simulink model "zCtr"  (Simulink 7.9)
settings: Solver=ode45  StartTime=0.0  StopTime=15  RelTol=1e-3
undefined symbols (not defined in the file): satThrust, sigbuilder_block
libraries: simulink x2
settings Model: Creator=userk  LastModifiedBy=userk

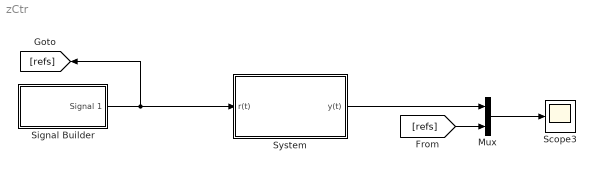
== system zCtr ==
  Mux : Mux  Inputs=2
  Scope3 : Scope
  Signal Builder : Subsystem  Tag=STV Subsys  LoadFcn=sigbuilder_block('load');  StartFcn=sigbuilder_block('start');  StopFcn=sigbuilder_block('stop');  ClipboardFcn=sigbuilder_block('clipboard');  mask(Sigbuilder block){}
      mask help: Simulink:masks:SigbuilderBlock_MD
      mask init:
      | if ~strcmp(get_param(bdroot(gcbh),'SimulationStatus'),'stopped') tuvar = sigbuilder_block('maskInit'); end
      settings: CopyFcn=sigbuilder_block('copy');  DeleteFcn=sigbuilder_block('delete');  ModelCloseFcn=sigbuilder_block('modelClose');  PreSaveFcn=sigbuilder_block('preSave');  PauseFcn=sigbuilder_block('pause');  ContinueFcn=sigbuilder_block('continue');  NameChangeFcn=sigbuilder_block('namechange');  OpenFcn=sigbuilder_block('open',[365.6 120.8 550.4 400 ]);  CloseFcn=sigbuilder_block('close');
      mask Display: plot(0, 0, 100, 100,[2, 2, 32, 32, 2], [68, 8, 8, 68, 68],[32, 2], [38, 38], [32, 19, 2],[53, 60, 44], [32, 17, 17, 2],[16, 16, 31, 31]);txt = getActiveGroup(gcbh);text(2, 100, txt,'verticalAlignment', 'top');
  System : Subsystem
  wires:
  Signal Builder/1(Signal 1) -> [refs], System/1(r(t))
  [refs] -> Mux/2
  Mux/1 -> Scope3/1
  System/1(y(t)) -> Mux/1

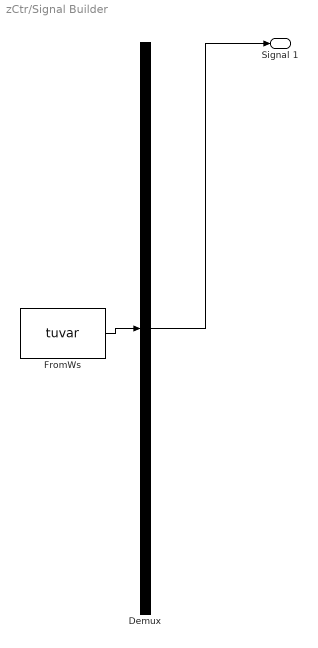
== system zCtr/Signal Builder ==
  Demux : Demux  Tag=STV Demux  Outputs=1
  FromWs : FromWorkspace  Tag=STV FromWs  VariableName=tuvar  SampleTime=0  SigBuilderData=DataTag0  VnvData=DataTag1
      SigBuilderData=|
      | common.afterFinalStr = 'Extrapolate'
      | common.sampleTime = 0
      | dataSet.timeRange = [0 10]
      | dataSet.name = 'Group 1'
      | sbobj.Groups.Name = 'Group 1'
      | sbobj.Groups.Signals.Name = 'Signal 1'
      | sbobj.Groups.Signals.XData = [0 4.06 4.06 6 6 10]
      | sbobj.Groups.Signals.YData = [0 0.995 1 1 0.995 0.01]
  Signal 1 : Outport  Tag=STV Outport
  wires:
  Demux/1 -> Signal 1/1
  FromWs/1 -> Demux/1

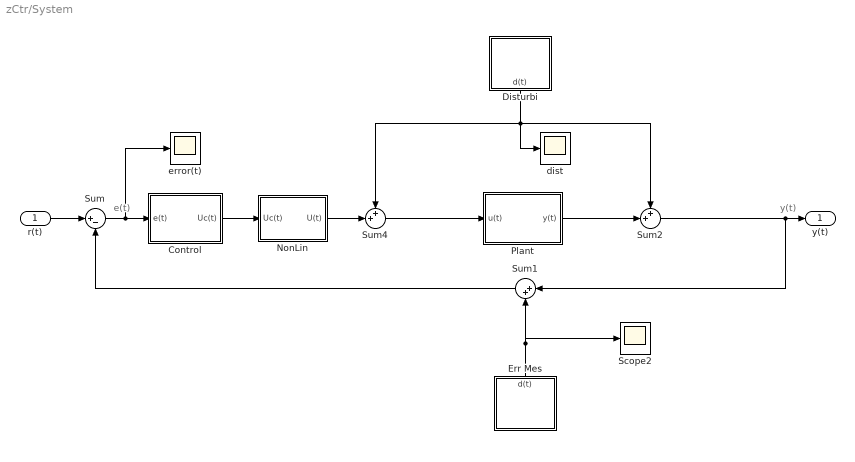
== system zCtr/System ==
  note: e(t)
  note: y(t)
  r(t) : Inport
  Control : Subsystem
  Disturbi : Subsystem
  Err Mes : Subsystem
  NonLin : Subsystem
  Plant : Subsystem
  Scope2 : Scope
      settings: SaveName=ScopeData2
  Sum : Sum  Inputs=|+-
  Sum1 : Sum  Inputs=|++
  Sum2 : Sum  Inputs=++|
  Sum4 : Sum  Inputs=++|
  dist : Scope
  error(t) : Scope
      settings: SaveName=ScopeData4
  y(t) : Outport
  wires:
  Sum/1 -> error(t)/1, Control/1(e(t))
  Plant/1(y(t)) -> Sum2/2
  Sum2/1 -> Sum1/1, y(t)/1
  Sum1/1 -> Sum/2
  Disturbi/1("  d(t)") -> dist/1, Sum4/1, Sum2/1
  Sum4/1 -> Plant/1(u(t))
  Control/1(Uc(t)) -> NonLin/1(Uc(t))
  NonLin/1(U(t)) -> Sum4/2
  r(t)/1 -> Sum/1
  Err Mes/1("  d(t)") -> Sum1/2, Scope2/1

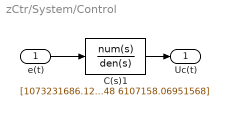
== system zCtr/System/Control ==
  e(t) : Inport
  C(s)1 : TransferFcn  Numerator=[1073231686.12918 1273486031.3238]  Denominator=[1 5043.9968441748 6107158.06951568]
  Uc(t) : Outport
  wires:
  e(t)/1 -> C(s)1/1
  C(s)1/1 -> Uc(t)/1

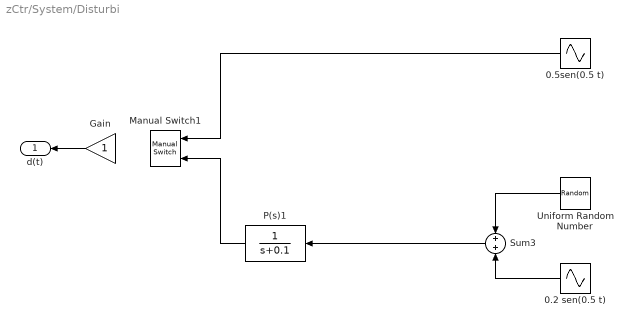
== system zCtr/System/Disturbi ==
  0.2 sen(0.5 t) : Sin  Amplitude=0.2  Frequency=0.5  Phase=1  SampleTime=0
  0.5sen(0.5 t) : Sin  Amplitude=0.5  Frequency=0.5  Phase=1  SampleTime=0
  Gain : Gain
  Manual Switch1 : simulink/Signal Routing/Manual Switch  sw=1  action=0  varsize=off
  P(s)1 : TransferFcn  Numerator=1  Denominator=[1 0.1]
  Sum3 : Sum
  Uniform Random Number : UniformRandomNumber  Minimum=-0.5  Maximum=0.5  SampleTime=0.1
  "  d(t)" : Outport
  wires:
  Uniform Random Number/1 -> Sum3/1
  0.2 sen(0.5 t)/1 -> Sum3/2
  Sum3/1 -> P(s)1/1
  0.5sen(0.5 t)/1 -> Manual Switch1/1
  P(s)1/1 -> Manual Switch1/2
  Gain/1 -> "  d(t)"/1

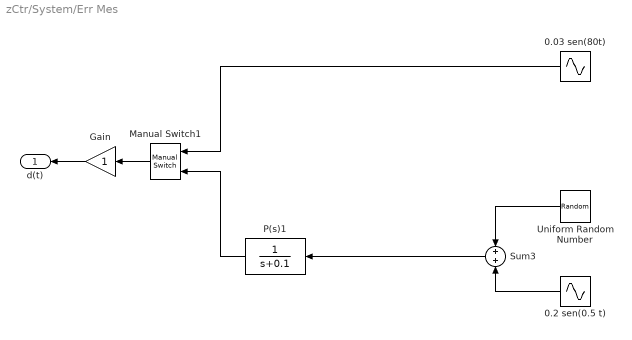
== system zCtr/System/Err Mes ==
  0.03 sen(80t) : Sin  Amplitude=0.003  Frequency=80  Phase=1  SampleTime=0
  0.2 sen(0.5 t) : Sin  Amplitude=0.02  Frequency=50  Phase=1  SampleTime=0
  Gain : Gain
  Manual Switch1 : simulink/Signal Routing/Manual Switch  sw=0  action=0  varsize=off
  P(s)1 : TransferFcn  Numerator=1  Denominator=[1 0.1]
  Sum3 : Sum
  Uniform Random Number : UniformRandomNumber  Minimum=-0.05  Maximum=0.05  SampleTime=0.1
  "  d(t)" : Outport
  wires:
  Uniform Random Number/1 -> Sum3/1
  0.2 sen(0.5 t)/1 -> Sum3/2
  Sum3/1 -> P(s)1/1
  0.03 sen(80t)/1 -> Manual Switch1/1
  P(s)1/1 -> Manual Switch1/2
  Gain/1 -> "  d(t)"/1
  Manual Switch1/1 -> Gain/1

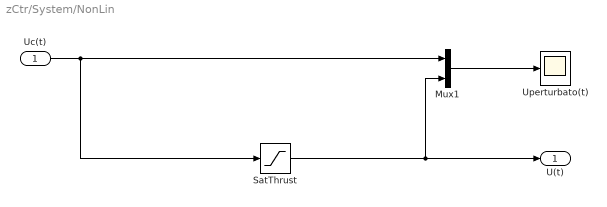
== system zCtr/System/NonLin ==
  Uc(t) : Inport
  Mux1 : Mux  Inputs=2
  SatThrust : Saturate  UpperLimit=satThrust  LowerLimit=-6
  Uperturbato(t) : Scope
      settings: ShowLegends=on  TimeRange=15  YMin=-150000  YMax=250000  SaveName=ScopeData5
  U(t) : Outport
  wires:
  Uc(t)/1 -> Mux1/1, SatThrust/1
  Mux1/1 -> Uperturbato(t)/1
  SatThrust/1 -> U(t)/1, Mux1/2

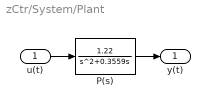
== system zCtr/System/Plant ==
  u(t) : Inport
  P(s) : TransferFcn  Numerator=1.22  Denominator=[1 0.3559 0]
  y(t) : Outport
  wires:
  u(t)/1 -> P(s)/1
  P(s)/1 -> y(t)/1
